simulink subsystem "RTB_FollowMobile"  (R2021b)
settings: Solver=VariableStepAuto  StartTime=0.0  StopTime=10.0  RelTol=1e-3
undefined symbols (not defined in the file): DiscIntNeverNeededParam, Earth, WGS84
libraries: aerolibtransform2 x1, mbdriLib x1, simulink x1
settings Model: Creator=promero  LastModifiedBy=promero

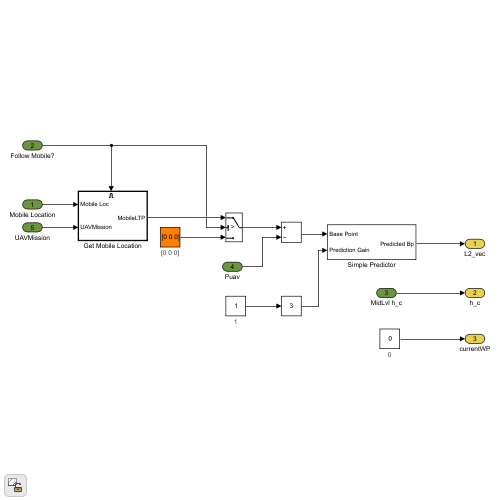
[thumbnail: Simulink's stored preview of the top-level diagram]
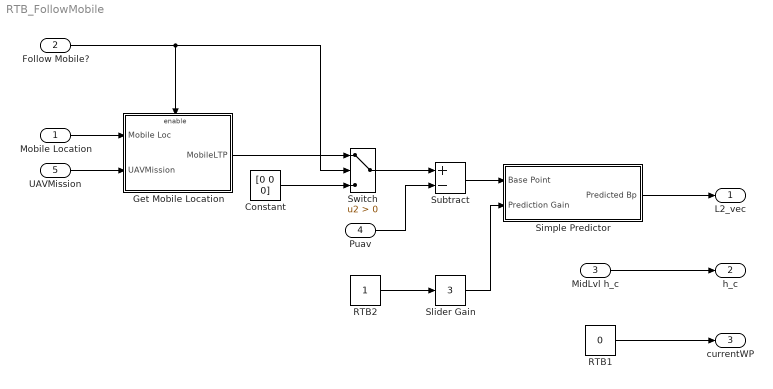
== system RTB_FollowMobile ==
  Mobile Location : Inport  RequirementInfo={} %GIDa_ca35f940_e1ad_42e7_941b_10536c388fbe
  Follow Mobile? : Inport  RequirementInfo={} %GIDa_ad13e8dc_ec9a_47f0_80b7_7d0d1963f418  Port=2
  MidLvl h_c : Inport  RequirementInfo={} %GIDa_bd4f81e6_dd43_4267_84cb_33e8203ec50d  Port=3
  Puav : Inport  RequirementInfo={} %GIDa_5cbd4891_6483_4116_8525_94c05fe1dada  Port=4
  UAVMission : Inport  RequirementInfo={} %GIDa_3f1e1908_9b00_4c30_bb01_fbaca6ca6f18  Port=5
  Constant : Constant  RequirementInfo={} %GIDa_4e21ae81_155e_43a7_b107_4e4a3d52644f  Value=[0 0 0]
      settings: AttributesFormatString=%<Value>
  Get Mobile Location : Subsystem  RequirementInfo={} %GIDa_b6066756_2761_48b1_a3ae_0cd13c0d4ffe
  RTB1 : Constant  RequirementInfo={} %GIDa_1b8e3493_d6d8_4b20_8e4b_3d811eacd586  Value=0  OutDataTypeStr=uint8
      settings: AttributesFormatString=%<Value>
  RTB2 : Constant  RequirementInfo={} %GIDa_08ccccfb_f4c9_4248_a413_0cdd4313bbc0
      settings: AttributesFormatString=%<Value>
  Simple Predictor : Subsystem  RequirementInfo={} %GIDa_1d535347_c4e5_43cd_ab72_815608b30cb9
  Slider Gain : simulink/Math Operations/Slider Gain  gain=3  low=1  high=20
  Subtract : Sum  RequirementInfo={} %GIDa_5a7f9c85_44dc_497f_9e81_a8319e7dc6b5  Inputs=+-
  Switch : Switch  RequirementInfo={} %GIDa_5ec98e65_a3e9_4858_a5c0_4a626262e4f2  Criteria=u2 > Threshold
  L2_vec : Outport  RequirementInfo={} %GIDa_365f03ca_933a_4a1d_8867_5c6fc7edcc17  VectorParamsAs1DForOutWhenUnconnected=off
  h_c : Outport  RequirementInfo={} %GIDa_8f4b6539_a1c8_48a5_af21_0f48be82863f  Port=2  VectorParamsAs1DForOutWhenUnconnected=off
  currentWP : Outport  RequirementInfo={} %GIDa_bfd815de_f018_4904_90dd_07b587f870a1  Port=3  VectorParamsAs1DForOutWhenUnconnected=off
  wires:
  Slider Gain/1 -> Simple Predictor/2(Prediction Gain)
  Mobile Location/1 -> Get Mobile Location/1(Mobile Loc)
  Switch/1 -> Subtract/1
  Simple Predictor/1(Predicted Bp) -> L2_vec/1
  MidLvl h_c/1 -> h_c/1
  Follow Mobile?/1 -> Switch/2, Get Mobile Location/Enable
  Puav/1 -> Subtract/2
  UAVMission/1 -> Get Mobile Location/2(UAVMission)
  Subtract/1 -> Simple Predictor/1(Base Point)
  RTB2/1 -> Slider Gain/1
  Get Mobile Location/1(MobileLTP) -> Switch/1
  Constant/1 -> Switch/3
  RTB1/1 -> currentWP/1

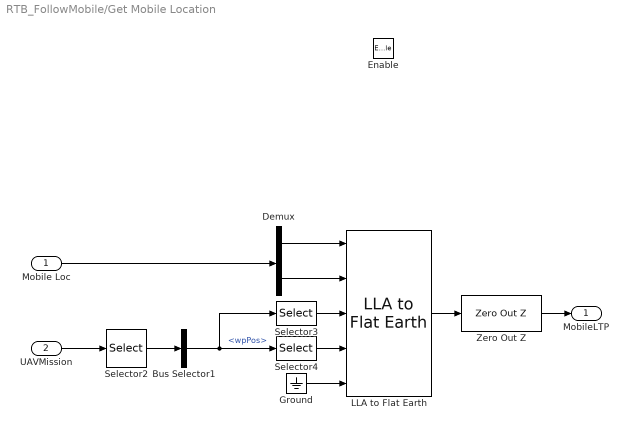
== system RTB_FollowMobile/Get Mobile Location ==
  Mobile Loc : Inport  RequirementInfo={} %GIDa_ec6e843b_ad91_4795_97fb_4c9383877dda
  UAVMission : Inport  RequirementInfo={} %GIDa_f52da48a_e533_4680_b2cc_bf60b651b338  Port=2
  Enable : EnablePort  RequirementInfo={} %GIDa_190d701b_0ec4_41b5_ba28_da66a5fc64bd
  Bus Selector1 : BusSelector  RequirementInfo={} %GIDa_83cf6588_55e0_4e7b_a276_1bf91a36057a  OutputSignals=wpPos
  Demux : Demux  RequirementInfo={} %GIDa_451641bf_41e0_44d1_859d_9203925e01a6  Outputs=[2 1]
  Ground : Ground  RequirementInfo={} %GIDa_386b5b47_598e_41d9_bf3c_e12464618da7
  LLA to Flat Earth : aerolibtransform2/LLA to Flat Earth  RequirementInfo={} %GIDa_303e6308_e4c9_43c4_a74b_1baede6ca5b7  units=Metric (MKS)  ptype=Earth (WGS84)  F=1/298.257223563  R=6378137  refPosPort=on  LL0=[0 10]  psi=0
      settings: SourceProductBaseCode=AE
  Selector2 : Selector  RequirementInfo={} %GIDa_be9654f5_b793_440e_87c9_728196b26158  InputPortWidth=10  IndexOptions=Index vector (dialog)  Indices=[1]  OutputSizes=1
  Selector3 : Selector  RequirementInfo={} %GIDa_4ed38eb1_77d3_482e_88b4_38f0b95b14b4  InputPortWidth=3  IndexOptions=Index vector (dialog)  Indices=[3]  OutputSizes=1
  Selector4 : Selector  RequirementInfo={} %GIDa_52a193f0_b950_4925_bd23_4924d6c01777  InputPortWidth=3  IndexOptions=Index vector (dialog)  Indices=[1 2]  OutputSizes=1
  Zero Out Z : mbdriLib/Utilities/Zero Out Z  RequirementInfo={} %GIDa_e5059f3c_e734_4c6a_85cd_33c275805bc8  SystemSampleTime=-1  VariantActivationTime=update diagram  Latency=0  AutoFrameSizeCalculation=off
  MobileLTP : Outport  RequirementInfo={} %GIDa_5d830e8d_38e9_45de_93b0_ae5dd504dca5  VectorParamsAs1DForOutWhenUnconnected=off
  wires:
  Ground/1 -> LLA to Flat Earth/5
  UAVMission/1 -> Selector2/1
  Demux/1 -> LLA to Flat Earth/1
  Selector3/1 -> LLA to Flat Earth/3
  Demux/2 -> LLA to Flat Earth/2
  Mobile Loc/1 -> Demux/1
  Selector2/1 -> Bus Selector1/1
  LLA to Flat Earth/1 -> Zero Out Z/1
  Selector4/1 -> LLA to Flat Earth/4
  Bus Selector1/1 -> Selector4/1, Selector3/1  "<wpPos>"
  Zero Out Z/1 -> MobileLTP/1

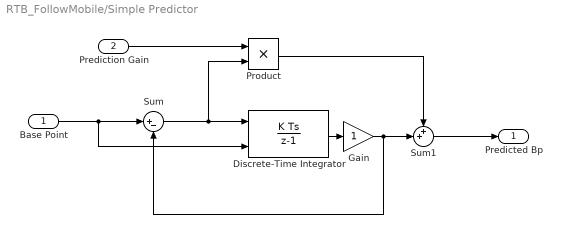
== system RTB_FollowMobile/Simple Predictor ==
  Base Point : Inport  RequirementInfo={} %GIDa_3220e753_9875_4e3c_85af_f9e384e5a573
  Prediction Gain : Inport  RequirementInfo={} %GIDa_dd14f0a6_3203_41b9_ac9a_d0daec642aa5  Port=2
  Discrete-Time Integrator : DiscreteIntegrator  RequirementInfo={} %GIDa_8eb1f3f8_d959_4c47_95b0_8ad939e2f606  InitialConditionSource=external  SampleTime=-1  ICPrevOutput=DiscIntNeverNeededParam  ICPrevScaledInput=DiscIntNeverNeededParam
  Gain : Gain  RequirementInfo={} %GIDa_7841b216_4a83_494c_974f_676de6825e54
      settings: AttributesFormatString=%<Gain>
  Product : Product  RequirementInfo={} %GIDa_bf227265_b8be_4610_baf9_0e5255d9d4b1  RndMeth=Zero
  Sum : Sum  RequirementInfo={} %GIDa_43a08168_5fd2_4758_ab75_8fe713b238d4  Inputs=|+-
  Sum1 : Sum  RequirementInfo={} %GIDa_afd1f304_5748_4145_86ac_d10c941a24ba  Inputs=++|
  Predicted Bp : Outport  RequirementInfo={} %GIDa_73632a73_5ec3_4a05_859f_9836d13e0d5a  VectorParamsAs1DForOutWhenUnconnected=off
  wires:
  Discrete-Time Integrator/1 -> Gain/1
  Sum/1 -> Discrete-Time Integrator/1, Product/2
  Gain/1 -> Sum/2, Sum1/2
  Product/1 -> Sum1/1
  Base Point/1 -> Sum/1, Discrete-Time Integrator/2
  Sum1/1 -> Predicted Bp/1
  Prediction Gain/1 -> Product/1
